simulink model "lab3b"  (R2022b)
settings: Solver=FixedStepAuto  StartTime=0.0  StopTime=1.0  FixedStep=1/1024  RelTol=1e-3
values from neighbouring files (symbols this model uses):
  amp = i    [lab3a.m]    (also in lab3a_script.m = db2mag(cur_pow); lab3bscript.m)
undefined symbols (not defined in the file or in its folder): lutdata, lutix
settings Model: Creator=simja  LastModifiedBy=simja
settings DataIOCC: ReturnWorkspaceOutputs=off

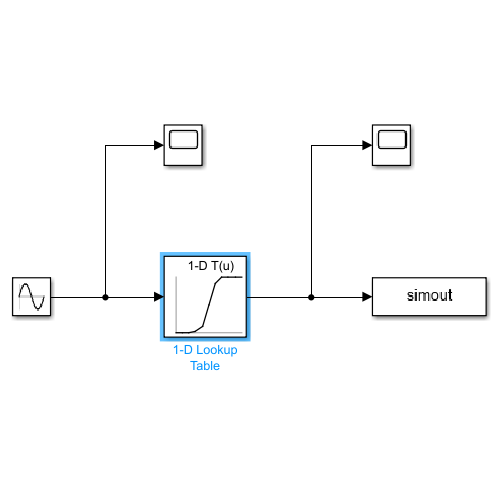
[thumbnail: Simulink's stored preview of the top-level diagram]
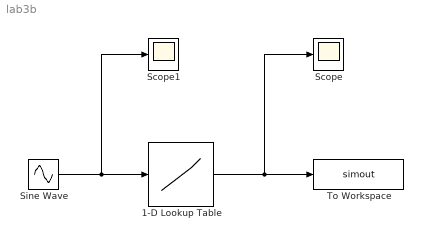
== system lab3b ==
  1-D Lookup Table : Lookup_n-D  NumberOfTableDimensions=1  BreakpointsForDimension1=lutix(2^10)  Table=lutdata(2^10)  InternalRulePriority=Speed  RndMeth=Simplest
  Scope : Scope
  Scope1 : Scope
  Sine Wave : Sin  Amplitude=amp  Frequency=2*5*pi  SampleTime=0
  To Workspace : ToWorkspace  VariableName=simout  SaveFormat=Structure With Time  SampleTime=-1
  wires:
  Sine Wave/1 -> Scope1/1, 1-D Lookup Table/1
  1-D Lookup Table/1 -> Scope/1, To Workspace/1
